simulink model "Laba2"  (R2022a)
settings: Solver=VariableStepAuto  StartTime=0.0  StopTime=10.0  RelTol=1e-3
settings Model: Creator=38098  LastModifiedBy=38098

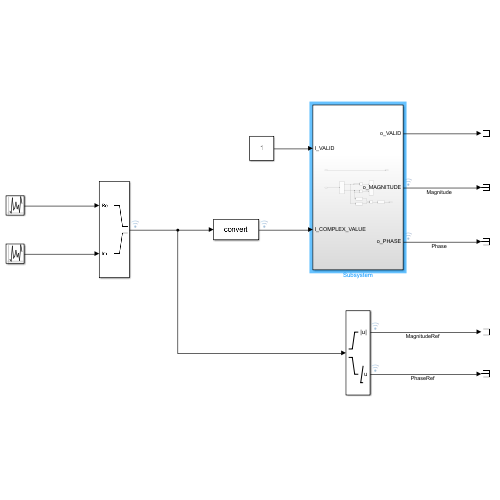
[thumbnail: Simulink's stored preview of the top-level diagram]
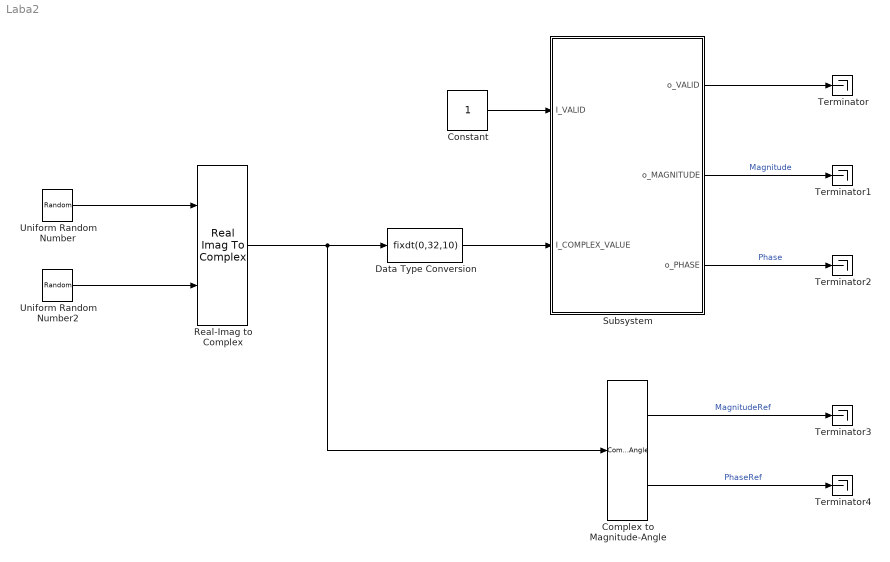
== system Laba2 ==
  Complex to Magnitude-Angle : ComplexToMagnitudeAngle
  Constant : Constant  OutDataTypeStr=boolean
  Data Type Conversion : DataTypeConversion  OutDataTypeStr=fixdt(0,32,10)  RndMeth=Round  SaturateOnIntegerOverflow=off
  Real-Imag to Complex : RealImagToComplex
  Subsystem : Subsystem
  Terminator{,1..4} (5 alike) : Terminator
  Uniform Random Number : UniformRandomNumber  Minimum=0  Maximum=2^(22)-1  Seed=22  SampleTime=1
  Uniform Random Number2 : UniformRandomNumber  Minimum=0  Maximum=2^(22)-1  Seed=23  SampleTime=1
  wires:
  Uniform Random Number/1 -> Real-Imag to Complex/1
  Uniform Random Number2/1 -> Real-Imag to Complex/2
  Real-Imag to Complex/1 -> Complex to Magnitude-Angle/1, Data Type Conversion/1
  Complex to Magnitude-Angle/1 -> Terminator3/1  "MagnitudeRef"
  Complex to Magnitude-Angle/2 -> Terminator4/1  "PhaseRef"
  Constant/1 -> Subsystem/1(I_VALID)
  Data Type Conversion/1 -> Subsystem/2(I_COMPLEX_VALUE)
  Subsystem/1(o_VALID) -> Terminator/1
  Subsystem/2(o_MAGNITUDE) -> Terminator1/1  "Magnitude"
  Subsystem/3(o_PHASE) -> Terminator2/1  "Phase"

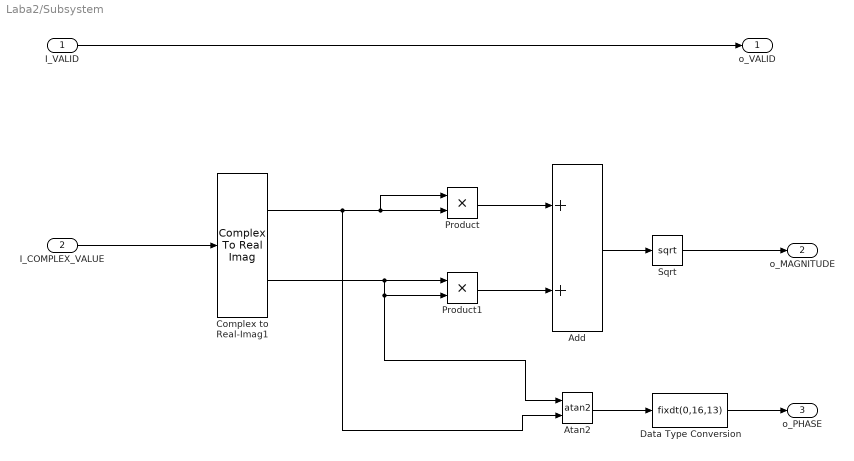
== system Laba2/Subsystem ==
  I_VALID : Inport
  I_COMPLEX_VALUE : Inport  Port=2
  Add : Sum  AccumDataTypeStr=fixdt(0,65,20)  OutDataTypeStr=fixdt(0,65,20)
  Atan2 : Trigonometry  Operator=atan2  ApproximationMethod=CORDIC
  Complex to Real-Imag1 : ComplexToRealImag
  Data Type Conversion : DataTypeConversion  OutDataTypeStr=fixdt(0,16,13)  RndMeth=Round  SaturateOnIntegerOverflow=off
  Product : Product
  Product1 : Product
  Sqrt : Sqrt  OutDataTypeStr=Inherit: Inherit via internal rule
  o_VALID : Outport
  o_MAGNITUDE : Outport  Port=2
  o_PHASE : Outport  Port=3
  wires:
  Product/1 -> Add/1
  Atan2/1 -> Data Type Conversion/1
  Add/1 -> Sqrt/1
  I_VALID/1 -> o_VALID/1
  Product1/1 -> Add/2
  I_COMPLEX_VALUE/1 -> Complex to Real-Imag1/1
  Sqrt/1 -> o_MAGNITUDE/1
  Data Type Conversion/1 -> o_PHASE/1
  Complex to Real-Imag1/2 -> Product1/1, Atan2/1, Product1/2
  Complex to Real-Imag1/1 -> Atan2/2, Product/1, Product/2
